simulink subsystem "heat_exchanger"  (R2024b)
settings: Solver=VariableStepAuto  StartTime=0.0  StopTime=10.0  RelTol=1e-3
model mask{U=1000, A=100}
  mask prompts: U "Thermal exchange coefficient [W/(m2.K)]"; A "Thermal exchange area [m2]"
settings Model: Creator=nerotb  LastModifiedBy=nerotb

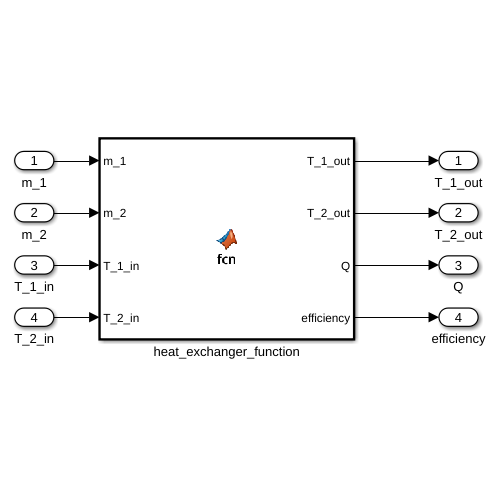
[thumbnail: Simulink's stored preview of the top-level diagram]
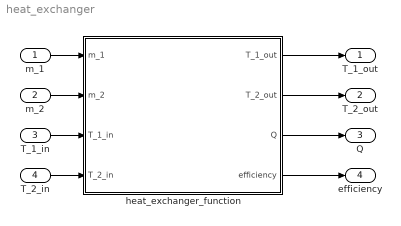
== system heat_exchanger ==
  m_1 : Inport
  m_2 : Inport  Port=2
  T_1_in : Inport  Port=3
  T_2_in : Inport  Port=4
  heat_exchanger_function : MATLAB Function  TreatAsAtomicUnit=on
  T_1_out : Outport
  T_2_out : Outport  Port=2
  Q : Outport  Port=3
  efficiency : Outport  Port=4
  wires:
  m_1/1 -> heat_exchanger_function/1(m_1)
  heat_exchanger_function/1(T_1_out) -> T_1_out/1
  T_2_in/1 -> heat_exchanger_function/4(T_2_in)
  T_1_in/1 -> heat_exchanger_function/3(T_1_in)
  m_2/1 -> heat_exchanger_function/2(m_2)
  heat_exchanger_function/2(T_2_out) -> T_2_out/1
  heat_exchanger_function/3(Q) -> Q/1
  heat_exchanger_function/4(efficiency) -> efficiency/1

== matlab function heat_exchanger/heat_exchanger_function ==
  data: m_1 input size=1; T_1_out output size=1; T_2_out output size=1; Q output size=1; m_2 input size=1; T_1_in input size=1; T_2_in input size=1; efficiency output size=1; U parameter size=1; A parameter size=1
function [T_1_out,T_2_out,Q, efficiency] = fcn(m_1, m_2, T_1_in, T_2_in, U, A)

    %% Summary
    % This function models a thermal heat exchanger. 
    % Flow 1 can be either cooled or warmed, depening on the sign of T_1_in - T_2_in
    %
    %% Model
    % This is base on the NTU method. Computation order:
    %   1. NTU
    %   2. Efficiency
    %   3. One of the output temperature
    %   4. Exchanged thermal power
    %   5. The other output temperature
    %
    %% Limitations
    % 1. This model does not take into account delays of propagation of the
    % flows in the heat exchanger. I.e.: it is supposed that a flow
    % entering at temperature T_1_in at macro time step t will exit at
    % temperature T_1_out also at time step t, no matter the value of m_1. 
    % 2. This model does not take into account thermal inertia of the heat
    % exchanger (e.g. inertia of steel)
    %
    %% Input variables
    % m_1 = mass flow on side 1 [kg/s]
    % m_2 = mass flow on side 2 [kg/s]
    % T_1_in = Input temperature on side 1 [K]
    % T_2_in = Input temperature on side 2 [K]

    %% Parameters
    % U = global thermal exchange coefficient [W/(K.m2)]
    % A = thermal exchange area [m2]
    
    %% Output variables
    % efficiency = heat exchanger efficiency [-]
    % T_1_out = Output temperature on side 1 [K]
    % T_2_out = Output temperature on side 2 [K]
    % Q = Exchanged thermal power [W]
    

    Cp_1 = 4180;
    Cp_2 = 4180;
    
    if m_2 <= 0 || m_1 <= 0 || T_1_in == T_2_in
        % trivial case : zero mass flows or equal input temperatures
        efficiency = 1;
        T_2_out = T_2_in;
        T_1_out = T_1_in;
        Q = 0;
    else
        % NTU computation
        C_min = min(m_1 * Cp_1, m_2 * Cp_2);
        C_max = max(m_1 * Cp_1, m_2 * Cp_2);
        C_r = C_min / C_max;
        NTU = U*A/C_min;
        % efficiency computation
        if C_r < 1
            As = exp(-NTU*(1-C_r));      % numerically stable computation
            efficiency = (1-As)/(1-As*C_r);
        else         
            % C_r == 1
            efficiency = NTU/(NTU+1);                  
        end

        F_min = min(Cp_1*m_1,Cp_2*m_2);
        T_2_out = T_2_in + (F_min/(Cp_2*m_2))*efficiency*(T_1_in - T_2_in); % same expression whether flow 2 is warmed up or cooled down
        Q = Cp_2*m_2*(T_2_out-T_2_in);
        T_1_out = T_1_in - Q / (m_1 * Cp_1);
    end
 


end
